simulink model "Xilanh"  (R2017b)
settings: Solver=VariableStepAuto  StartTime=0.0  StopTime=400  RelTol=1e-3
libraries: simulink x1
settings Model: Creator=win7  LastModifiedBy=windy

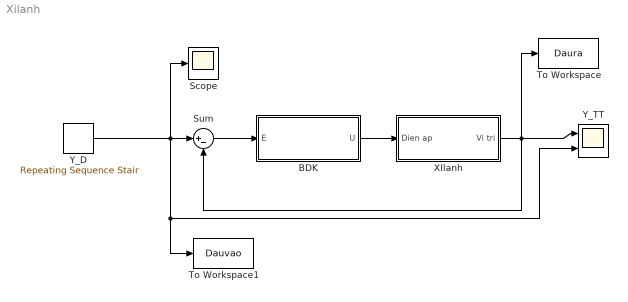
== system Xilanh ==
  BDK : Subsystem
  Scope : Scope
  Sum : Sum  Inputs=|+-
  To Workspace : ToWorkspace  VariableName=Daura  SaveFormat=Structure With Time  SampleTime=-1
  To Workspace1 : ToWorkspace  VariableName=Dauvao  SaveFormat=Structure With Time  SampleTime=-1
  XIlanh : Subsystem
  Y_D : simulink/Sources/Repeating Sequence Stair  OutValues=[15 25 10].'  tsamp=50  OutMin=[]  OutMax=[]  OutDataTypeStr=double  OutputDataTypeScalingMode=double  OutDataType=fixdt(0,8)  ConRadixGroup=Best Precision: Vector-wise  OutScaling=2^-12
  Y_TT : Scope  NumInputPorts=2
  wires:
  Sum/1 -> BDK/1(E)
  BDK/1(U) -> XIlanh/1(Dien ap)
  XIlanh/1(Vi tri) -> To Workspace/1, Y_TT/1, Sum/2
  Y_D/1 -> Y_TT/2, To Workspace1/1, Scope/1, Sum/1

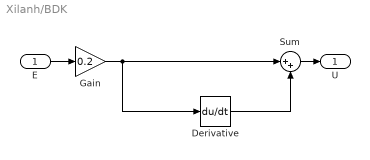
== system Xilanh/BDK ==
  E : Inport
  Derivative : Derivative
  Gain : Gain  Gain=0.2
  Sum : Sum  Inputs=|++
  U : Outport
  wires:
  E/1 -> Gain/1
  Sum/1 -> U/1
  Gain/1 -> Derivative/1, Sum/1
  Derivative/1 -> Sum/2

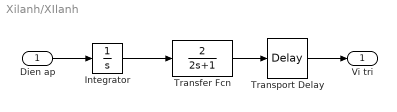
== system Xilanh/XIlanh ==
  Dien ap : Inport
  Integrator : Integrator
  Transfer Fcn : TransferFcn  Numerator=[2]  Denominator=[2 1]
  Transport Delay : TransportDelay  DelayTime=0.2
  Vi tri : Outport
  wires:
  Dien ap/1 -> Integrator/1
  Integrator/1 -> Transfer Fcn/1
  Transport Delay/1 -> Vi tri/1
  Transfer Fcn/1 -> Transport Delay/1
